simulink model "example_House_Simple_ISOgm_CONF"  (R2013b)
settings: Solver=ode45  StartTime=0.0  StopTime=365*24*3600  RelTol=1e-3
libraries: carnot x4
settings Model: Creator=drhf  LastModifiedBy=drhf
settings OptimizationCC: ExpressionDepthLimit=2147483647
settings DebuggingCC: StateNameClashWarn=warning
settings GRTTargetCC: CombineOutputUpdateFcns=off  GRTInterface=on

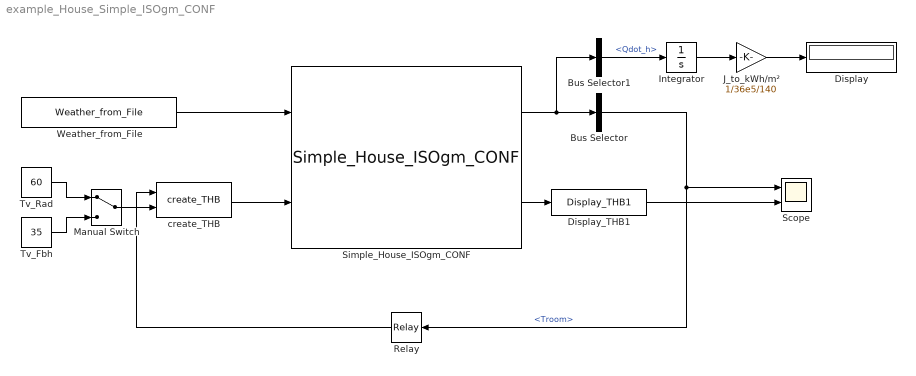
== system example_House_Simple_ISOgm_CONF ==
  Bus Selector : BusSelector  OutputSignals=Troom
  Bus Selector1 : BusSelector  OutputSignals=Qdot.Qdot_h
  Display : Display
  Display_THB1 : carnot/Outputs/Display_THB1  t=off  m=on  p=off  id=off  mix=off  d=off
  Integrator : Integrator
  J_to_kWh/m² : Gain  Gain=1/36e5/140
  Manual Switch : ManualSwitch
  Relay : Relay  OnSwitchValue=20.1  OffSwitchValue=19.9  OnOutputValue=0  OffOutputValue=800/3600
  Scope : Scope  NumInputPorts=2
      settings: YMin=19.75~0  YMax=24.75~0.225
  Simple_House_ISOgm_CONF : carnot/Load/Houses/Simple_House_ISOgm_CONF  parameterfile=Default_SimpleHouseISOgm  tini=20
  Tv_Fbh : Constant  Value=35
  Tv_Rad : Constant  Value=60
  Weather_from_File : carnot/Weather/Weather_from_File  file=DE_TRY2010_04_averageYear  ext=.mat
  create_THB : carnot/Source/Simple/create_THB  p=1e5  fluid=Water  mix=0  dia=0.02  mID=No Pressure Drop
  wires:
  Bus Selector/1 -> Scope/1, Relay/1  "<Troom>"
  Relay/1 -> create_THB/1
  Weather_from_File/1 -> Simple_House_ISOgm_CONF/1
  create_THB/1 -> Simple_House_ISOgm_CONF/2
  Simple_House_ISOgm_CONF/1 -> Bus Selector/1, Bus Selector1/1
  Simple_House_ISOgm_CONF/2 -> Display_THB1/1
  Display_THB1/1 -> Scope/2
  Bus Selector1/1 -> Integrator/1  "<Qdot_h>"
  Integrator/1 -> J_to_kWh/m²/1
  J_to_kWh/m²/1 -> Display/1
  Manual Switch/1 -> create_THB/2
  Tv_Rad/1 -> Manual Switch/1
  Tv_Fbh/1 -> Manual Switch/2
